simulink model "navin_model"  (R2025b)
settings: Solver=ode45  StartTime=0.0  StopTime=1180  RelTol=1e-4
undefined symbols (not defined in the file): cycle, vehicle
libraries: slpidlib x1, simulink x1
settings Model: Creator=Piyush  LastModifiedBy=Piyush

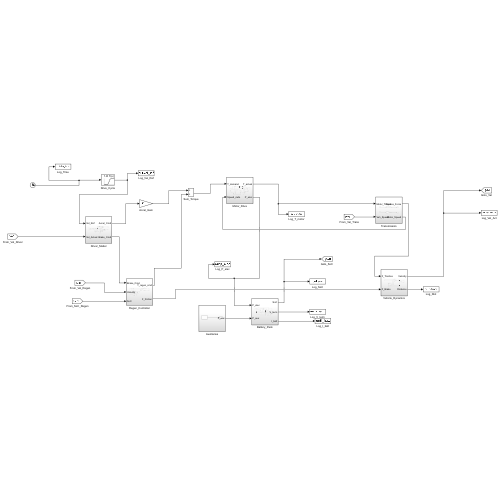
[thumbnail: Simulink's stored preview of the top-level diagram]
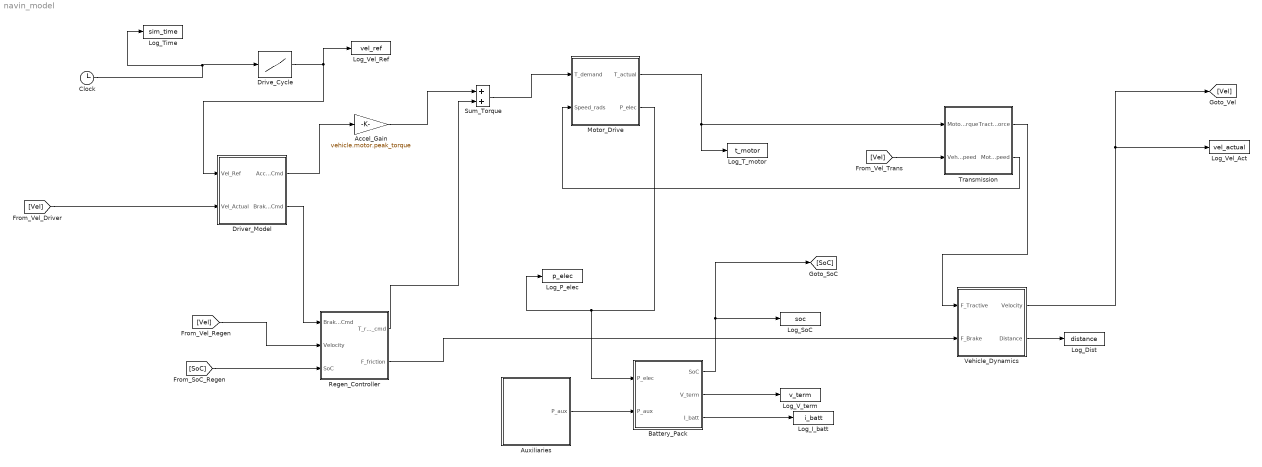
== system navin_model ==
  Accel_Gain : Gain  Gain=vehicle.motor.peak_torque
  Auxiliaries : Subsystem
  Battery_Pack : Subsystem
  Clock : Clock
  Drive_Cycle : Lookup_n-D  NumberOfTableDimensions=1  BreakpointsForDimension1=cycle.time  Table=cycle.velocity_ms  InternalRulePriority=Speed  RndMeth=Simplest
  Driver_Model : Subsystem
  Log_Dist : ToWorkspace  VariableName=distance  SaveFormat=Structure With Time  SampleTime=-1
  Log_I_batt : ToWorkspace  VariableName=i_batt  SaveFormat=Structure With Time  SampleTime=-1
  Log_P_elec : ToWorkspace  VariableName=p_elec  SaveFormat=Structure With Time  SampleTime=-1
  Log_SoC : ToWorkspace  VariableName=soc  SaveFormat=Structure With Time  SampleTime=-1
  Log_T_motor : ToWorkspace  VariableName=t_motor  SaveFormat=Structure With Time  SampleTime=-1
  Log_Time : ToWorkspace  VariableName=sim_time  SampleTime=-1
  Log_V_term : ToWorkspace  VariableName=v_term  SaveFormat=Structure With Time  SampleTime=-1
  Log_Vel_Act : ToWorkspace  VariableName=vel_actual  SaveFormat=Structure With Time  SampleTime=-1
  Log_Vel_Ref : ToWorkspace  VariableName=vel_ref  SaveFormat=Structure With Time  SampleTime=-1
  Motor_Drive : Subsystem
  Regen_Controller : Subsystem
  Sum_Torque : Sum
  Transmission : Subsystem
  Vehicle_Dynamics : Subsystem
  wires:
  Clock/1 -> Drive_Cycle/1, Log_Time/1
  Drive_Cycle/1 -> Log_Vel_Ref/1, Driver_Model/1(Vel_Ref)
  Driver_Model/2(Brake_Cmd) -> Regen_Controller/1(Brake_Cmd)
  Driver_Model/1(Accel_Cmd) -> Accel_Gain/1
  Accel_Gain/1 -> Sum_Torque/1
  Regen_Controller/1(T_regen_cmd) -> Sum_Torque/2
  Sum_Torque/1 -> Motor_Drive/1(T_demand)
  Transmission/2(Motor_Speed) -> Motor_Drive/2(Speed_rads)
  Motor_Drive/1(T_actual) -> Log_T_motor/1, Transmission/1(Motor_Torque)
  Transmission/1(Tractive_Force) -> Vehicle_Dynamics/1(F_Tractive)
  Regen_Controller/2(F_friction) -> Vehicle_Dynamics/2(F_Brake)
  Motor_Drive/2(P_elec) -> Log_P_elec/1, Battery_Pack/1(P_elec)
  Auxiliaries/1(P_aux) -> Battery_Pack/2(P_aux)
  Vehicle_Dynamics/1(Velocity) -> [Vel], Log_Vel_Act/1
  [Vel] -> Driver_Model/2(Vel_Actual)
  [Vel] -> Regen_Controller/2(Velocity)
  [Vel] -> Transmission/2(Veh_Speed)
  Battery_Pack/1(SoC) -> [SoC], Log_SoC/1
  [SoC] -> Regen_Controller/3(SoC)
  Battery_Pack/2(V_term) -> Log_V_term/1
  Battery_Pack/3(I_batt) -> Log_I_batt/1
  Vehicle_Dynamics/2(Distance) -> Log_Dist/1

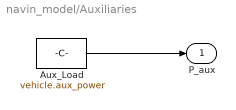
== system navin_model/Auxiliaries ==
  Aux_Load : Constant  Value=vehicle.aux_power
  P_aux : Outport
  wires:
  Aux_Load/1 -> P_aux/1

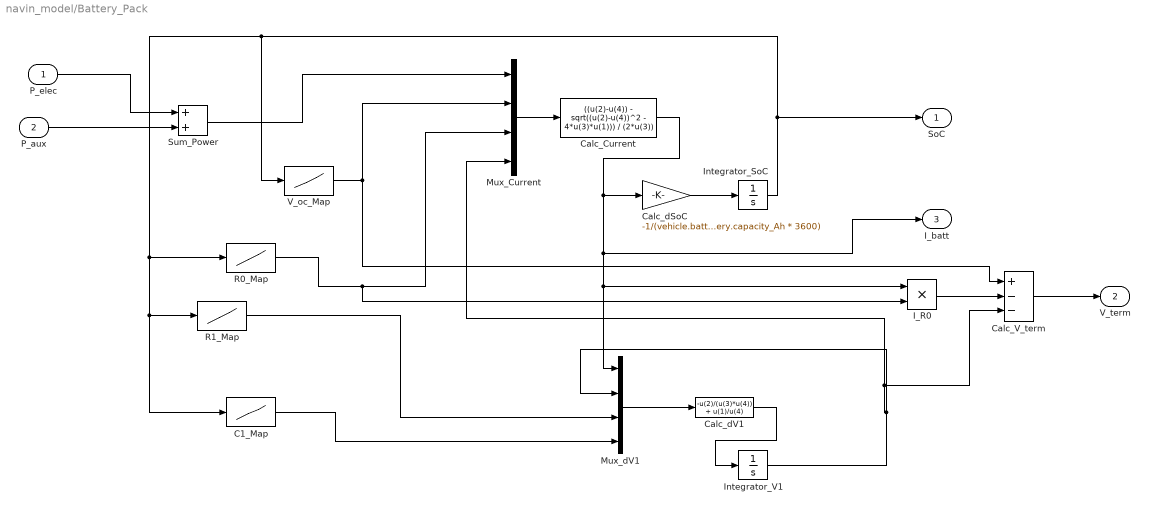
== system navin_model/Battery_Pack ==
  P_elec : Inport
  P_aux : Inport  Port=2
  C1_Map : Lookup_n-D  NumberOfTableDimensions=1  BreakpointsForDimension1=vehicle.battery.soc_vec  Table=vehicle.battery.c1_vec  InternalRulePriority=Speed  RndMeth=Simplest
  Calc_Current : Fcn  Expr=((u(2)-u(4)) - sqrt((u(2)-u(4))^2 - 4*u(3)*u(1))) / (2*u(3))
  Calc_V_term : Sum  Inputs=+--
  Calc_dSoC : Gain  Gain=-1/(vehicle.battery.capacity_Ah * 3600)
  Calc_dV1 : Fcn  Expr=-u(2)/(u(3)*u(4)) + u(1)/u(4)
  I_R0 : Product
  Integrator_SoC : Integrator  InitialCondition=1
  Integrator_V1 : Integrator
  Mux_Current : Mux
  Mux_dV1 : Mux
  R0_Map : Lookup_n-D  NumberOfTableDimensions=1  BreakpointsForDimension1=vehicle.battery.soc_vec  Table=vehicle.battery.r0_vec  InternalRulePriority=Speed  RndMeth=Simplest
  R1_Map : Lookup_n-D  NumberOfTableDimensions=1  BreakpointsForDimension1=vehicle.battery.soc_vec  Table=vehicle.battery.r1_vec  InternalRulePriority=Speed  RndMeth=Simplest
  Sum_Power : Sum
  V_oc_Map : Lookup_n-D  NumberOfTableDimensions=1  BreakpointsForDimension1=vehicle.battery.soc_vec  Table=vehicle.battery.ocv_vec  InternalRulePriority=Speed  RndMeth=Simplest
  SoC : Outport
  V_term : Outport  Port=2
  I_batt : Outport  Port=3
  wires:
  P_elec/1 -> Sum_Power/1
  P_aux/1 -> Sum_Power/2
  Sum_Power/1 -> Mux_Current/1
  V_oc_Map/1 -> Calc_V_term/1, Mux_Current/2
  R0_Map/1 -> Mux_Current/3, I_R0/2
  Mux_Current/1 -> Calc_Current/1
  Calc_Current/1 -> Mux_dV1/1, I_R0/1, I_batt/1, Calc_dSoC/1
  R1_Map/1 -> Mux_dV1/3
  C1_Map/1 -> Mux_dV1/4
  Mux_dV1/1 -> Calc_dV1/1
  Calc_dV1/1 -> Integrator_V1/1
  Integrator_V1/1 -> Mux_Current/4, Calc_V_term/3, Mux_dV1/2
  Calc_dSoC/1 -> Integrator_SoC/1
  Integrator_SoC/1 -> SoC/1, C1_Map/1, R1_Map/1, R0_Map/1, V_oc_Map/1
  I_R0/1 -> Calc_V_term/2
  Calc_V_term/1 -> V_term/1

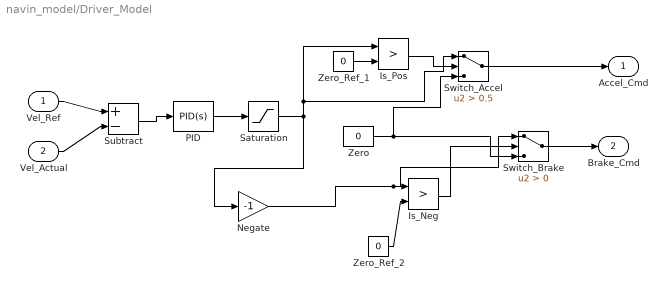
== system navin_model/Driver_Model ==
  Vel_Ref : Inport
  Vel_Actual : Inport  Port=2
  Is_Neg : RelationalOperator  Operator=>  OutDataTypeStr=boolean  RndMeth=Simplest  InputSameDT=off
  Is_Pos : RelationalOperator  Operator=>  OutDataTypeStr=boolean  RndMeth=Simplest  InputSameDT=off
  Negate : Gain  Gain=-1
  PID : slpidlib/PID Controller  Controller=PID  Form=Parallel  TimeDomain=Continuous-time  UseExternalTs=off  SampleTime=-1  IntegratorMethod=Forward Euler  FilterMethod=Forward Euler  ControllerParametersSource=internal  P=vehicle.driver.Kp  I=vehicle.driver.Ki  UseKiTs=off  D=0  UseExternalDerivativeSource=off  N=100  UseFilter=on  TunerSelectOption=Transfer Function Based (PID Tuner App)  InitialConditionSource=internal  InitialConditionForIntegrator=0  InitialConditionForFilter=0  DifferentiatorICPrevScaledInput=0  ExternalReset=none  TrackingMode=off  Kt=1  LimitOutput=off  SatLimitsSource=internal  UpperSaturationLimit=inf  LowerSaturationLimit=-inf  LinearizeAsGain=on  AntiWindupMode=none  Kb=1  LimitIntegrator=off  UpperIntegratorSaturationLimit=inf  LowerIntegratorSaturationLimit=-inf  POutMin=[]  POutMax=[]  IOutMin=[]  IOutMax=[]  DOutMin=[]  DOutMax=[]  NOutMin=[]  NOutMax=[]  SumOutMin=[]  SumOutMax=[]  SaturationOutMin=[]  SaturationOutMax=[]  PParamMin=[]  PParamMax=[]  IParamMin=[]  IParamMax=[]  DParamMin=[]  DParamMax=[]  NParamMin=[]  NParamMax=[]  KbParamMin=[]  KbParamMax=[]  KtParamMin=[]  KtParamMax=[]  KbOutMin=[]  KbOutMax=[]  KtOutMin=[]  KtOutMax=[]  IntegratorOutMin=[]  IntegratorOutMax=[]  FilterOutMin=[]  FilterOutMax=[]  SumI1OutMin=[]  SumI1OutMax=[]  SumI2OutMin=[]  SumI2OutMax=[]  SumI3OutMin=[]  SumI3OutMax=[]  SumI4OutMin=[]  SumI4OutMax=[]  SumDOutMin=[]  SumDOutMax=[]  DifferentiatorOutMin=[]  DifferentiatorOutMax=[]  FilterDiffOutCoefMin=[]  FilterDiffOutCoefMax=[]  ReciprocalOutMin=[]  ReciprocalOutMax=[]  SumDenOutMin=[]  SumDenOutMax=[]  SumNumOutMin=[]  SumNumOutMax=[]  DivideOutMin=[]  DivideOutMax=[]  UdiffTsProdOutMin=[]  UdiffTsProdOutMax=[]  NTsProdOutMin=[]  NTsProdOutMax=[]  UintegralTsProdOutMin=[]  UintegralTsProdOutMax=[]  UngainTsProdOutMin=[]  UngainTsProdOutMax=[]  ClampingZeroOutDataTypeStr=Inherit: Inherit via back propagation  ClampingZeroOutMin=[]  ClampingZeroOutMax=[]  FilterDenConstantOutDataTypeStr=Inherit: Inherit via back propagation  FilterDenConstantOutMin=[]  FilterDenConstantOutMax=[]  PCopyOutDataTypeStr=Inherit: Inherit via back propagation  PCopyOutMin=[]  PCopyOutMax=[]  NCopyOutDataTypeStr=Inherit: Inherit via back propagation  NCopyOutMin=[]  NCopyOutMax=[]  IntegratorContinuousStateAttributes=''  IntegratorStateMustResolveToSignalObject=off  IntegratorRTWStateStorageClass=Auto  FilterContinuousStateAttributes=''  FilterStateMustResolveToSignalObject=off  FilterRTWStateStorageClass=Auto  ParallelPVariant=InternalParameters  IdealPVariant=Disabled  IVariant=InternalParameters  DVariant=InternalParameters  IntegratorVariant=Continuous  SatVariant=Disabled  AWVariant=Passthrough  PCopyVariant=Disabled  TRVariant=Disabled  FdbkBlocksVariant=Forward  IdealPFdbkVariant=Disabled  SatFdbkVariant=Disabled  DerivativeFilterVariant=ContFilter  NVariant=InternalParameters  NCopyVariant=Disabled  FilterICVariant=InternalICsFilter  IntegratorICVariant=InternalICs  ExternalResetVariant=Disabled  TRSumVariant=Passthrough  SumFdbkVariant=Disabled  SumVariant=Sum_PID  TsampFilterVariant=InternalTs  TsampNgainVariant=Passthrough  TsampIntegralVariant=Disabled_SignalSpec  ExternalSaturationOutDataTypeStr=Inherit: Same as second input  DerivativeSourceVariant=ErrorSignal  PreIntVariant=InternalPreInt
  Saturation : Saturate  UpperLimit=1  LowerLimit=-1
  Subtract : Sum  Inputs=+-
  Switch_Accel : Switch  Criteria=u2 > Threshold  Threshold=0.5  SaturateOnIntegerOverflow=off  InputSameDT=off
  Switch_Brake : Switch  Criteria=u2 > Threshold  SaturateOnIntegerOverflow=off  InputSameDT=off
  Zero : Constant  Value=0
  Zero_Ref_1 : Constant  Value=0
  Zero_Ref_2 : Constant  Value=0
  Accel_Cmd : Outport
  Brake_Cmd : Outport  Port=2
  wires:
  Vel_Ref/1 -> Subtract/1
  Vel_Actual/1 -> Subtract/2
  Subtract/1 -> PID/1
  PID/1 -> Saturation/1
  Saturation/1 -> Switch_Accel/1, Is_Pos/1, Negate/1
  Zero_Ref_1/1 -> Is_Pos/2
  Is_Pos/1 -> Switch_Accel/2
  Zero/1 -> Switch_Brake/3, Switch_Accel/3
  Negate/1 -> Is_Neg/1, Switch_Brake/1
  Zero_Ref_2/1 -> Is_Neg/2
  Is_Neg/1 -> Switch_Brake/2
  Switch_Accel/1 -> Accel_Cmd/1
  Switch_Brake/1 -> Brake_Cmd/1

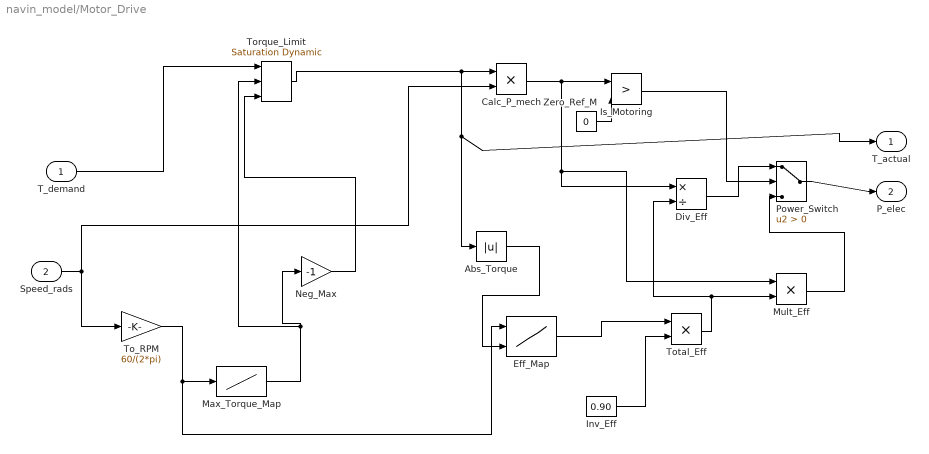
== system navin_model/Motor_Drive ==
  T_demand : Inport
  Speed_rads : Inport  Port=2
  Abs_Torque : Abs  SaturateOnIntegerOverflow=off
  Calc_P_mech : Product
  Div_Eff : Product  Inputs=*/
  Eff_Map : Lookup_n-D  BreakpointsForDimension1=vehicle.motor.speed_vec  BreakpointsForDimension2=vehicle.motor.torque_vec  Table=vehicle.motor.eff_map  InternalRulePriority=Speed  RndMeth=Simplest
      settings: InputPortMap=u0,u1
  Inv_Eff : Constant  Value=0.90
  Is_Motoring : RelationalOperator  Operator=>  OutDataTypeStr=boolean  RndMeth=Simplest  InputSameDT=off
  Max_Torque_Map : Lookup_n-D  NumberOfTableDimensions=1  BreakpointsForDimension1=vehicle.motor.speed_vec  Table=vehicle.motor.max_torque  InternalRulePriority=Speed  RndMeth=Simplest
  Mult_Eff : Product
  Neg_Max : Gain  Gain=-1
  Power_Switch : Switch  Criteria=u2 > Threshold  SaturateOnIntegerOverflow=off  InputSameDT=off
  To_RPM : Gain  Gain=60/(2*pi)
  Torque_Limit : simulink/Discontinuities/Saturation Dynamic  OutMin=[]  OutMax=[]  OutDataTypeStr=Inherit: Same as second input  OutDataType=fixdt(1, 16)  OutScaling=2^-10  DoSatur=off
  Total_Eff : Product
  Zero_Ref_M : Constant  Value=0
  T_actual : Outport
  P_elec : Outport  Port=2
  wires:
  Speed_rads/1 -> To_RPM/1, Calc_P_mech/2
  To_RPM/1 -> Max_Torque_Map/1, Eff_Map/1
  Max_Torque_Map/1 -> Neg_Max/1, Torque_Limit/2
  T_demand/1 -> Torque_Limit/1
  Neg_Max/1 -> Torque_Limit/3
  Torque_Limit/1 -> Abs_Torque/1, T_actual/1, Calc_P_mech/1
  Abs_Torque/1 -> Eff_Map/2
  Eff_Map/1 -> Total_Eff/1
  Inv_Eff/1 -> Total_Eff/2
  Calc_P_mech/1 -> Div_Eff/1, Mult_Eff/1, Is_Motoring/1
  Zero_Ref_M/1 -> Is_Motoring/2
  Total_Eff/1 -> Div_Eff/2, Mult_Eff/2
  Is_Motoring/1 -> Power_Switch/2
  Div_Eff/1 -> Power_Switch/1
  Mult_Eff/1 -> Power_Switch/3
  Power_Switch/1 -> P_elec/1

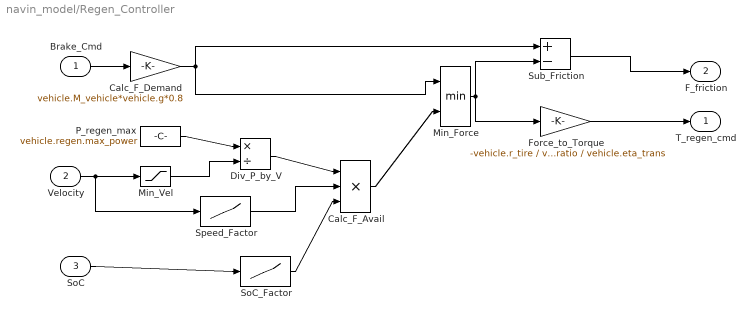
== system navin_model/Regen_Controller ==
  Brake_Cmd : Inport
  Velocity : Inport  Port=2
  SoC : Inport  Port=3
  Calc_F_Avail : Product  Inputs=3
  Calc_F_Demand : Gain  Gain=vehicle.M_vehicle*vehicle.g*0.8
  Div_P_by_V : Product  Inputs=*/
  Force_to_Torque : Gain  Gain=-vehicle.r_tire / vehicle.gear_ratio / vehicle.eta_trans
  Min_Force : MinMax  Inputs=2
  Min_Vel : Saturate  UpperLimit=inf  LowerLimit=0.1
  P_regen_max : Constant  Value=vehicle.regen.max_power
  SoC_Factor : Lookup_n-D  NumberOfTableDimensions=1  BreakpointsForDimension1=[0 0.9 0.98 1]  Table=[1 1 0 0]  InternalRulePriority=Speed  RndMeth=Simplest
  Speed_Factor : Lookup_n-D  NumberOfTableDimensions=1  BreakpointsForDimension1=[0 0.5 2.0 100]  Table=[0 0 1 1]  InternalRulePriority=Speed  RndMeth=Simplest
  Sub_Friction : Sum  Inputs=+-
  T_regen_cmd : Outport
  F_friction : Outport  Port=2
  wires:
  Brake_Cmd/1 -> Calc_F_Demand/1
  Velocity/1 -> Speed_Factor/1, Min_Vel/1
  P_regen_max/1 -> Div_P_by_V/1
  Min_Vel/1 -> Div_P_by_V/2
  SoC/1 -> SoC_Factor/1
  Div_P_by_V/1 -> Calc_F_Avail/1
  Speed_Factor/1 -> Calc_F_Avail/2
  SoC_Factor/1 -> Calc_F_Avail/3
  Calc_F_Demand/1 -> Min_Force/1, Sub_Friction/1
  Calc_F_Avail/1 -> Min_Force/2
  Min_Force/1 -> Sub_Friction/2, Force_to_Torque/1
  Force_to_Torque/1 -> T_regen_cmd/1
  Sub_Friction/1 -> F_friction/1

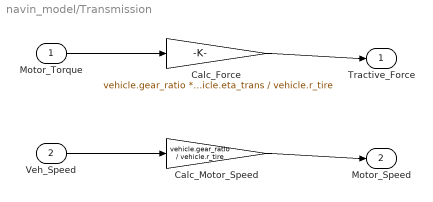
== system navin_model/Transmission ==
  Motor_Torque : Inport
  Veh_Speed : Inport  Port=2
  Calc_Force : Gain  Gain=vehicle.gear_ratio * vehicle.eta_trans / vehicle.r_tire
  Calc_Motor_Speed : Gain  Gain=vehicle.gear_ratio / vehicle.r_tire
  Tractive_Force : Outport
  Motor_Speed : Outport  Port=2
  wires:
  Motor_Torque/1 -> Calc_Force/1
  Veh_Speed/1 -> Calc_Motor_Speed/1
  Calc_Force/1 -> Tractive_Force/1
  Calc_Motor_Speed/1 -> Motor_Speed/1

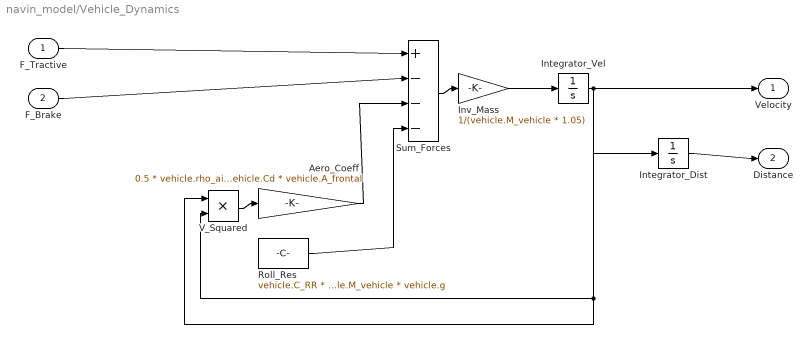
== system navin_model/Vehicle_Dynamics ==
  F_Tractive : Inport
  F_Brake : Inport  Port=2
  Aero_Coeff : Gain  Gain=0.5 * vehicle.rho_air * vehicle.Cd * vehicle.A_frontal
  Integrator_Dist : Integrator
  Integrator_Vel : Integrator
  Inv_Mass : Gain  Gain=1/(vehicle.M_vehicle * 1.05)
  Roll_Res : Constant  Value=vehicle.C_RR * vehicle.M_vehicle * vehicle.g
  Sum_Forces : Sum  Inputs=+---
  V_Squared : Product
  Velocity : Outport
  Distance : Outport  Port=2
  wires:
  V_Squared/1 -> Aero_Coeff/1
  F_Tractive/1 -> Sum_Forces/1
  F_Brake/1 -> Sum_Forces/2
  Aero_Coeff/1 -> Sum_Forces/3
  Roll_Res/1 -> Sum_Forces/4
  Sum_Forces/1 -> Inv_Mass/1
  Inv_Mass/1 -> Integrator_Vel/1
  Integrator_Vel/1 -> V_Squared/1, V_Squared/2, Integrator_Dist/1, Velocity/1
  Integrator_Dist/1 -> Distance/1
